simulink model "P2_SIL_Model_Diag"  (R2016a)
settings: Solver=ode2  StartTime=0.0  StopTime=Cycle_End  RelTol=1e-3
undefined symbols (not defined in the file): air, APP1_OOR, APP2_OOR, APP_Conversion_IN, APP_Mismatch, bms_inletair_temp, bms_maxchargecurrent, bms_maxdischargecurrent, BMS_Notfallkuehlung, BPP_Flt, cal, clt, ClutchEngag, CrankRequest, dcdc, eng, Engine, EngOverTemp, ENGTRQ_MSMCH_Degraded_CP, ENGTRQ_MSMCH_ErrCritical_CP, ENGTRQ_MSMCH_LimpHome_CP, EngTrqMismatch, env, ess, ESS, ESSOverTemp, fd, FFD, g, gb, Grade, IMG, KeyPos_Flt, KeyPosition, lib_APP_Conversion_IN, lib_ESS_plant_V1_2, lib_OBC_Manager, LossCAN, max_vehicle_rad_air_flow, MCUOverTemp, mot, MotDirMismatch, MotOverTemp, MotTrqMismatch, mph2kph, mph2ms, NeutralGear, obc, OBC_Manager, ParkGear, PRNDL_Flt, ReverseGear, RFD, rho, ShiftLeverPosition, sigbuilder_block, Speed, t_amb, time, tloop ... (+2)
libraries: simulink x104, EC2_libraries x12, Diagnostic x11, lib_CANerror_Detect x3, Utility x1
(part 5 of 11)

== system P2_SIL_Model_Diag/Plant Actuators/CAN/HV_CAN/BMS_Hybrid ==
  In1 : Inport
  Bus Selector : BusSelector  OutputSignals=BMS_CAN.BMS_Plugin
  Out1 : Outport
  wires:
  Bus Selector/1 -> Out1/1  "<BMS_Plugin>"
  In1/1 -> Bus Selector/1

== system P2_SIL_Model_Diag/Plant Actuators/CAN/HV_CAN/MCU ==
  In1 : Inport
  Bus Selector : BusSelector  OutputSignals=MCU_CAN
  Out1 : Outport
  wires:
  Bus Selector/1 -> Out1/1  "<MCU_CAN>"
  In1/1 -> Bus Selector/1

== system P2_SIL_Model_Diag/Plant Actuators/CAN/HV_CAN/OBC ==
  In1 : Inport
  Bus Selector : BusSelector  OutputSignals=OBC_CAN
  Out1 : Outport
  wires:
  Bus Selector/1 -> Out1/1  "<OBC_CAN>"
  In1/1 -> Bus Selector/1

== system P2_SIL_Model_Diag/Plant Actuators/CAN/VEH_CAN/BCM ==
  In1 : Inport
  Out1 : Outport
  wires:
  In1/1 -> Out1/1

== system P2_SIL_Model_Diag/Plant Actuators/CAN/VEH_CAN/EBCM ==
  In1 : Inport
  Out1 : Outport
  wires:
  In1/1 -> Out1/1

== system P2_SIL_Model_Diag/Plant Actuators/CAN/VEH_CAN/ICCM ==
  In1 : Inport
  Out1 : Outport
  wires:
  In1/1 -> Out1/1

== system P2_SIL_Model_Diag/Plant Actuators/CAN/VEH_CAN/TCM ==
  In1 : Inport
  Out1 : Outport
  wires:
  In1/1 -> Out1/1

== system P2_SIL_Model_Diag/Plant Sensors/CAN/EBCAN/BMS_Antrieb ==
  In1 : Inport
  Bus Selector : BusSelector  OutputSignals=to_EBCAN.ISO_Funktionaler_Req_All
  Out1 : Outport
  wires:
  Bus Selector/1 -> Out1/1  "<ISO_Funktionaler_Req_All>"
  In1/1 -> Bus Selector/1

== system P2_SIL_Model_Diag/Plant Sensors/CAN/EBCAN/ECM ==
  In1 : Inport
  Bus Selector : BusSelector  OutputSignals=to_EBCAN.ECM_CAN
  Out1 : Outport
  wires:
  Bus Selector/1 -> Out1/1  "<ECM_CAN>"
  In1/1 -> Bus Selector/1

== system P2_SIL_Model_Diag/Plant Sensors/CAN/HV_CAN/APM ==
  In1 : Inport
  Bus Selector : BusSelector  OutputSignals=to_HV_CAN.to_APM
  Out1 : Outport
  wires:
  In1/1 -> Bus Selector/1
  Bus Selector/1 -> Out1/1  "<to_APM>"

== system P2_SIL_Model_Diag/Plant Sensors/CAN/HV_CAN/BMS_Hybrid ==
  In1 : Inport
  Bus Selector : BusSelector  OutputSignals=to_HV_CAN.to_BMS_Hybrid
  Out1 : Outport
  wires:
  Bus Selector/1 -> Out1/1  "<to_BMS_Hybrid>"
  In1/1 -> Bus Selector/1

== system P2_SIL_Model_Diag/Plant Sensors/CAN/HV_CAN/MCU ==
  In1 : Inport
  Bus Selector : BusSelector  OutputSignals=to_HV_CAN.to_MCU
  Out1 : Outport
  wires:
  Bus Selector/1 -> Out1/1  "<to_MCU>"
  In1/1 -> Bus Selector/1

== system P2_SIL_Model_Diag/Plant Sensors/CAN/HV_CAN/OBC ==
  In1 : Inport
  Bus Selector : BusSelector  OutputSignals=to_HV_CAN.to_OBC
  Out1 : Outport
  wires:
  Bus Selector/1 -> Out1/1  "<to_OBC>"
  In1/1 -> Bus Selector/1

== system P2_SIL_Model_Diag/Plant Sensors/CAN/VEH_CAN/BCM ==
  In1 : Inport
  Bus Selector : BusSelector  OutputSignals=to_VEH_CAN.HAct_to_BCM
  Out1 : Outport
  wires:
  Bus Selector/1 -> Out1/1  "<HAct_to_BCM>"
  In1/1 -> Bus Selector/1

== system P2_SIL_Model_Diag/Plant Sensors/CAN/VEH_CAN/EBCM ==
  In1 : Inport
  Bus Selector : BusSelector  OutputSignals=to_VEH_CAN.HAct_to_EBCM
  Out1 : Outport
  wires:
  Bus Selector/1 -> Out1/1  "<HAct_to_EBCM>"
  In1/1 -> Bus Selector/1

== system P2_SIL_Model_Diag/Plant Sensors/CAN/VEH_CAN/ICCM ==
  In1 : Inport
  Bus Selector : BusSelector  OutputSignals=to_VEH_CAN.HAct_to_ICCM
  Out1 : Outport
  wires:
  Bus Selector/1 -> Out1/1  "<HAct_to_ICCM>"
  In1/1 -> Bus Selector/1

== system P2_SIL_Model_Diag/Plant Sensors/CAN/VEH_CAN/TCM ==
  In1 : Inport
  Bus Selector : BusSelector  OutputSignals=to_VEH_CAN.HAct_to_TCM
  Out1 : Outport
  wires:
  Bus Selector/1 -> Out1/1  "<HAct_to_TCM>"
  In1/1 -> Bus Selector/1

== system P2_SIL_Model_Diag/Sensors/Analog/APP Manipulation/APP1_Conversion ==
  APP1_IN : Inport
  APP1_IN_Max : Constant  Value=cal.APP1.IN_Max
  APP1_IN_Max_SC : Constant  Value=cal.APP.IN_Max_SC
  APP1_IN_Min : Constant  Value=cal.APP1.IN_Min
  Constant : Constant  Value=0
  Divide : Product  Inputs=*/
  Gain : Gain  Gain=100
  Relational Operator : RelationalOperator  Operator=>  OutDataTypeStr=boolean
  Sum1 : Sum  Inputs=|+-
  Sum2 : Sum  Inputs=|-+
  Sum3 : Sum  Inputs=|++
  Switch1 : Switch  Threshold=1
  APP1 : Outport
  OOR : Outport  Port=2
  wires:
  Sum3/1 -> Relational Operator/2
  Switch1/1 -> APP1/1
  APP1_IN_Max_SC/1 -> Sum3/2
  Relational Operator/1 -> Switch1/2, OOR/1  "APP1_SC_Fault"
  Constant/1 -> Switch1/1
  Gain/1 -> Switch1/3
  Divide/1 -> Gain/1
  Sum2/1 -> Divide/2
  Sum1/1 -> Divide/1
  APP1_IN/1 -> Relational Operator/1, Sum1/1
  APP1_IN_Max/1 -> Sum3/1, Sum2/2
  APP1_IN_Min/1 -> Sum1/2, Sum2/1

== system P2_SIL_Model_Diag/Sensors/Analog/APP Manipulation/APP2_Conversion ==
  APP2_IN : Inport
  APP1_IN_Max_SC : Constant  Value=cal.APP.IN_Max_SC
  APP2_IN_Max : Constant  Value=cal.APP2.IN_Max
  APP2_IN_Min : Constant  Value=cal.APP2.IN_Min
  Constant : Constant  Value=0
  Divide : Product  Inputs=*/
  Gain1 : Gain  Gain=100
  Relational Operator : RelationalOperator  Operator=>  OutDataTypeStr=boolean
  Sum1 : Sum  Inputs=|++
  Sum2 : Sum  Inputs=|+-
  Sum3 : Sum  Inputs=|-+
  Switch1 : Switch  Threshold=1
  APP2 : Outport
  OOR : Outport  Port=2
  wires:
  Switch1/1 -> APP2/1
  APP1_IN_Max_SC/1 -> Sum1/2
  Sum1/1 -> Relational Operator/2
  Relational Operator/1 -> Switch1/2, OOR/1  "APP2_SC_Fault"
  Constant/1 -> Switch1/1
  Gain1/1 -> Switch1/3
  Divide/1 -> Gain1/1
  Sum3/1 -> Divide/2
  Sum2/1 -> Divide/1
  APP2_IN/1 -> Relational Operator/1, Sum2/1
  APP2_IN_Max/1 -> Sum1/1, Sum3/2
  APP2_IN_Min/1 -> Sum2/2, Sum3/1

== system P2_SIL_Model_Diag/Sensors/CAN/EBCAN/BMS_Antrieb ==
  In1 : Inport
  Bus Creator : BusCreator  Inputs=2
  Bus Selector : BusSelector  OutputSignals=NMH_BMS
  ISO_Hybrid_01_Resp : Subsystem
  NMH_BMS : Subsystem
  Out1 : Outport
  wires:
  In1/1 -> Bus Selector/1
  Bus Selector/1 -> NMH_BMS/1(In1)  "<NMH_BMS>"
  NMH_BMS/1(Out1) -> Bus Creator/1
  ISO_Hybrid_01_Resp/1(Out1) -> Bus Creator/2
  Bus Creator/1 -> Out1/1

== system P2_SIL_Model_Diag/Sensors/CAN/EBCAN/CCM ==
  In1 : Inport
  ISO_Hybrid_01_Resp : Subsystem
  NMH_BMS : Subsystem
  Out1 : Outport

== system P2_SIL_Model_Diag/Sensors/CAN/EBCAN/ECM ==
  In1 : Inport
  Bus Creator : BusCreator  Inputs=7
  Bus Selector : BusSelector  OutputSignals=Sensors_to_ECM.EngActStdyStTorq_Nm,Sensors_to_ECM.EngSpd_RPM,ECM_to_Actuators.VehSpdAvgDrvn,ECM_to_Actuators.EngRunAtv,ECM_to_Actuators.EngTrqCmd,ECM_to_Actuators.Eng_Temp,ECM_to_Actuators.ECM_RollingAliveCnt
  ETEI_Engine_Torque_Status : Subsystem
  PPEI_Vehicle_Speed_and_Distance : Subsystem
  Out1 : Outport
  wires:
  In1/1 -> Bus Selector/1
  Bus Selector/1 -> ETEI_Engine_Torque_Status/1(In1)  "<EngActStdyStTorq_Nm>"
  Bus Selector/2 -> Bus Creator/2  "<EngSpd_RPM>"
  Bus Selector/3 -> PPEI_Vehicle_Speed_and_Distance/1(In1)  "<VehSpdAvgDrvn>"
  ETEI_Engine_Torque_Status/1(Out1) -> Bus Creator/1
  PPEI_Vehicle_Speed_and_Distance/1(Out1) -> Bus Creator/3
  Bus Creator/1 -> Out1/1
  Bus Selector/4 -> Bus Creator/4  "<EngRunAtv>"
  Bus Selector/5 -> Bus Creator/5  "<EngTrqCmd>"
  Bus Selector/6 -> Bus Creator/6  "<Eng_Temp>"
  Bus Selector/7 -> Bus Creator/7  "<ECM_RollingAliveCnt>"

== system P2_SIL_Model_Diag/Sensors/CAN/HV_CAN/APM ==
  In1 : Inport
  Out1 : Outport
  wires:
  In1/1 -> Out1/1

== system P2_SIL_Model_Diag/Sensors/CAN/HV_CAN/BMS_Hybrid ==
  In1 : Inport
  BMS_HYB_02 : Subsystem
  BMS_HYB_03 : Subsystem
  BMS_HYB_04 : Subsystem
  Bus Creator : BusCreator  Inputs=5
  Bus Selector : BusSelector  OutputSignals=BMS_HYB_02,BMS_HYB_04,BMS_HYB_03,RollingAliveCnt,BMS_HYB_06
  Out1 : Outport
  wires:
  In1/1 -> Bus Selector/1
  Bus Selector/1 -> BMS_HYB_02/1(In1)  "<BMS_HYB_02>"
  Bus Selector/2 -> BMS_HYB_04/1(In1)  "<BMS_HYB_04>"
  Bus Creator/1 -> Out1/1
  BMS_HYB_02/1(Out1) -> Bus Creator/1
  BMS_HYB_04/1(Out1) -> Bus Creator/2
  Bus Selector/3 -> BMS_HYB_03/1(In1)  "<BMS_HYB_03>"
  BMS_HYB_03/1(Out1) -> Bus Creator/3
  Bus Selector/4 -> Bus Creator/4  "<RollingAliveCnt>"
  Bus Selector/5 -> Bus Creator/5  "<BMS_HYB_06>"

== system P2_SIL_Model_Diag/Sensors/CAN/HV_CAN/MCU ==
  note: torque feedback should be from sensors, not MCU to Actuators
      | in this model, mot_torq_out and MotTrqFdbck are the same signals
  In1 : Inport
  Bus Creator : BusCreator  Inputs=11
  Bus Selector : BusSelector  OutputSignals=Sensors_to_MCU.mot_spd_out,Sensors_to_MCU.mot_crr_out,MCU_to _Actuator.InverterEnabled,Sensors_to_MCU.mot_volt_in,Sensors_to_MCU.mot_temp,MCU_to _Actuator.Torque_Command,MCU_to _Actuator.MotTrqFdbck,MCU_to _Actuator.EngageClutch,Sensors_to_MCU.mcu_temp,MCU_to _Actuator.RollingAliveCnt,Sensors_to_MCU.clt_plant_spd_in
  M165_Motor_Position_Info : Subsystem
  M166_Current_Info : Subsystem
  M167_Voltage_Info : Subsystem
  M170_Internal_States : Subsystem
  M172_Torque_And_Timer_Info : Subsystem
  M192_Command_Message : Subsystem
  Out1 : Outport
  wires:
  In1/1 -> Bus Selector/1
  Bus Selector/1 -> M165_Motor_Position_Info/1(In1)  "<mot_spd_out>"
  Bus Selector/2 -> M166_Current_Info/1(In1)  "<mot_crr_out>"
  Bus Selector/3 -> M170_Internal_States/1(In1)  "<InverterEnabled>"
  M165_Motor_Position_Info/1(Out1) -> Bus Creator/1
  M166_Current_Info/1(Out1) -> Bus Creator/2
  M170_Internal_States/1(Out1) -> Bus Creator/3
  Bus Creator/1 -> Out1/1
  Bus Selector/5 -> Bus Creator/5  "<mot_temp>"
  Bus Selector/6 -> M192_Command_Message/1(In1)  "<Torque_Command>"
  Bus Selector/7 -> M172_Torque_And_Timer_Info/1(In1)  "<MotTrqFdbck>"
  Bus Selector/4 -> M167_Voltage_Info/1(In1)  "<mot_volt_in>"
  M167_Voltage_Info/1(Out1) -> Bus Creator/4
  M192_Command_Message/1(Out1) -> Bus Creator/6
  M172_Torque_And_Timer_Info/1(Out1) -> Bus Creator/7
  Bus Selector/8 -> Bus Creator/8  "<EngageClutch>"
  Bus Selector/9 -> Bus Creator/9  "<mcu_temp>"
  Bus Selector/10 -> Bus Creator/10  "<RollingAliveCnt>"
  Bus Selector/11 -> Bus Creator/11  "<clt_plant_spd_in>"

== system P2_SIL_Model_Diag/Sensors/CAN/HV_CAN/OBC ==
  In1 : Inport
  Out1 : Outport
  wires:
  In1/1 -> Out1/1

== system P2_SIL_Model_Diag/Sensors/CAN/VEH_CAN/BCM ==
  In1 : Inport
  Bus Creator : BusCreator  Inputs=2
  Bus Selector : BusSelector  OutputSignals=SysPwrMd,BrkPdlPos
  PPEI_Brake_Apply_Status : Subsystem
  PPEI_Platfrom_General_Status : Subsystem
  Out1 : Outport
  wires:
  In1/1 -> Bus Selector/1
  Bus Selector/1 -> PPEI_Platfrom_General_Status/1(In1)  "<SysPwrMd>"
  Bus Selector/2 -> PPEI_Brake_Apply_Status/1(In1)  "<BrkPdlPos>"
  PPEI_Platfrom_General_Status/1(Out1) -> Bus Creator/1
  PPEI_Brake_Apply_Status/1(Out1) -> Bus Creator/2
  Bus Creator/1 -> Out1/1

== system P2_SIL_Model_Diag/Sensors/CAN/VEH_CAN/EBCM ==
  In1 : Inport
  PPEI_Chassis_General_Status_1 : Subsystem
  Out1 : Outport
  wires:
  PPEI_Chassis_General_Status_1/1(Out1) -> Out1/1

== system P2_SIL_Model_Diag/Sensors/CAN/VEH_CAN/ICCM ==
  In1 : Inport
  Out1 : Outport
  wires:
  In1/1 -> Out1/1

== system P2_SIL_Model_Diag/Sensors/CAN/VEH_CAN/TCM ==
  In1 : Inport
  Bus Creator : BusCreator  Inputs=3
  Bus Selector : BusSelector  OutputSignals=TCM_to _Actuator.TransEstGear,TCM_to _Actuator.LockupCmd,TCM_to _Actuator.TrnsShftLvrPos
  Out1 : Outport
  wires:
  In1/1 -> Bus Selector/1
  Bus Selector/1 -> Bus Creator/1  "<TransEstGear>"
  Bus Selector/2 -> Bus Creator/2  "<LockupCmd>"
  Bus Selector/3 -> Bus Creator/3  "<TrnsShftLvrPos>"
  Bus Creator/1 -> Out1/1

== system P2_SIL_Model_Diag/Camaro Plant Model/ESS/ESS/ESSThermal/LowerLimit ==
  In : Inport
  Constant : Constant  Value=Lolimit
  MinMax : MinMax  Function=max  Inputs=2
  Out : Outport
  wires:
  Constant/1 -> MinMax/2
  In/1 -> MinMax/1
  MinMax/1 -> Out/1

== system P2_SIL_Model_Diag/Camaro Plant Model/ESS/ESS/ESSThermal/LowerLimit1 ==
  In : Inport
  Constant : Constant  Value=Lolimit
  MinMax : MinMax  Function=max  Inputs=2
  Out : Outport
  wires:
  Constant/1 -> MinMax/2
  In/1 -> MinMax/1
  MinMax/1 -> Out/1

== system P2_SIL_Model_Diag/Camaro Plant Model/ESS/ESS/LoadCharacteristics/LowerLimit1 ==
  In : Inport
  Constant : Constant  Value=Lolimit
  MinMax : MinMax  Function=max  Inputs=2
  Out : Outport
  wires:
  Constant/1 -> MinMax/2
  In/1 -> MinMax/1
  MinMax/1 -> Out/1

== system P2_SIL_Model_Diag/Camaro Plant Model/ESS/ESS/LoadCharacteristics/LowerLimit2 ==
  In : Inport
  Constant : Constant  Value=Lolimit
  MinMax : MinMax  Function=max  Inputs=2
  Out : Outport
  wires:
  Constant/1 -> MinMax/2
  In/1 -> MinMax/1
  MinMax/1 -> Out/1

== system P2_SIL_Model_Diag/Camaro Plant Model/ESS/ESS/LoadCharacteristics/SOC Calculation ==
  Current : Inport
  3600*nominal battery capacity : Constant  Value=3600*ess.plant.init.batcap
  Sum3 : Sum  Inputs=|++
  To Workspace : ToWorkspace  VariableName=ess_soc_percent_hist  SampleTime=-1
      settings: Decimation=WORKSPACE_DECIMATION
  i/3600C : Product  Inputs=*/  RndMeth=Zero
  soc previous state : Memory  X0=ess.plant.init.initial_soc/100  InheritSampleTime=on
  soc limits : Saturate  UpperLimit=1  LowerLimit=0
  tloop : Gain  Gain=tloop
  to % : Gain  Gain=100
  SOC : Outport
  wires:
  3600*nominal battery capacity/1 -> i/3600C/2  "As"
  i/3600C/1 -> tloop/1  "dSOC/s"
  to %/1 -> To Workspace/1
  soc limits/1 -> to %/1, SOC/1, soc previous state/1
  tloop/1 -> Sum3/1  "dSOC"
  Sum3/1 -> soc limits/1
  soc previous state/1 -> Sum3/2  "soc"
  Current/1 -> i/3600C/1  "A"

== system P2_SIL_Model_Diag/Camaro Plant Model/ESS/Soft BMS/Energy Consumption/Divide by zero ==
  In1 : Inport
  Compare To Constant : simulink/Logic and Bit Operations/Compare To Constant  relop===  const=0  OutDataTypeStr=boolean
  Constant1 : Constant  Value=eps
  Switch2 : Switch  Criteria=u2 > Threshold
  Out1 : Outport
  wires:
  Constant1/1 -> Switch2/1
  Compare To Constant/1 -> Switch2/2
  In1/1 -> Switch2/3, Compare To Constant/1
  Switch2/1 -> Out1/1

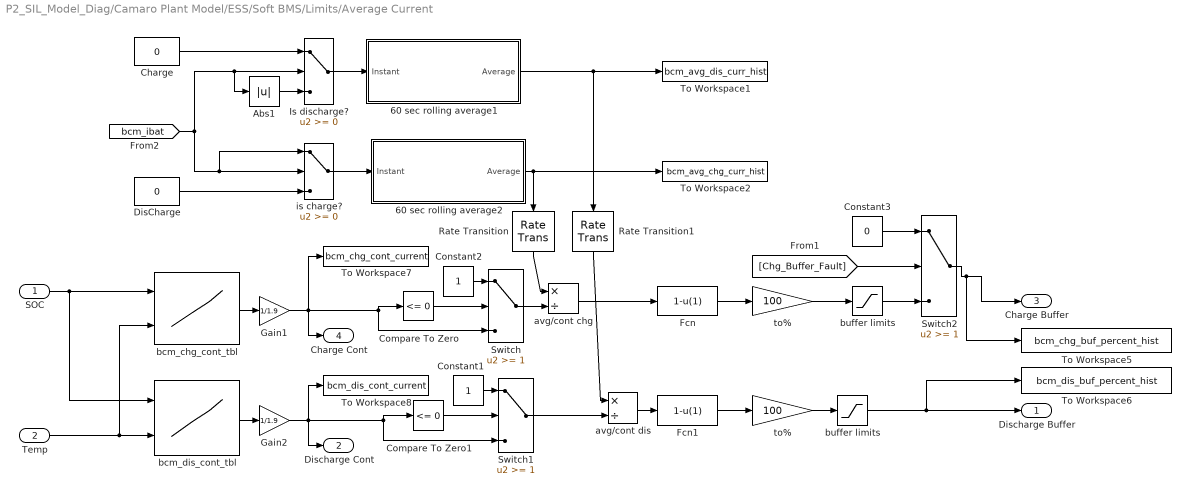
== system P2_SIL_Model_Diag/Camaro Plant Model/ESS/Soft BMS/Limits/Average Current ==
  SOC : Inport
  Temp : Inport  Port=2
  60 sec rolling average1 : Subsystem
  60 sec rolling average2 : Subsystem
  Abs1 : Abs
  Charge : Constant  Value=0
  Compare To Zero : simulink/Logic and Bit Operations/Compare To Zero  relop=<=  OutDataTypeStr=boolean
  Compare To Zero1 : simulink/Logic and Bit Operations/Compare To Zero  relop=<=  OutDataTypeStr=boolean
  Constant1 : Constant
  Constant2 : Constant
  Constant3 : Constant  Value=0
  DisCharge : Constant  Value=0
  Fcn : Fcn  Expr=1-u(1)
  Fcn1 : Fcn  Expr=1-u(1)
  Gain1 : Gain  Gain=1/1.9
  Gain2 : Gain  Gain=1/1.9
  Is discharge? : Switch
  Rate Transition : RateTransition
  Rate Transition1 : RateTransition
  Switch : Switch  Threshold=1
  Switch1 : Switch  Threshold=1
  Switch2 : Switch  Threshold=1
  To Workspace1 : ToWorkspace  VariableName=bcm_avg_dis_curr_hist  SampleTime=-1
      settings: Decimation=WORKSPACE_DECIMATION
  To Workspace2 : ToWorkspace  VariableName=bcm_avg_chg_curr_hist  SampleTime=-1
      settings: Decimation=WORKSPACE_DECIMATION
  To Workspace5 : ToWorkspace  VariableName=bcm_chg_buf_percent_hist  SampleTime=-1
      settings: Decimation=WORKSPACE_DECIMATION
  To Workspace6 : ToWorkspace  VariableName=bcm_dis_buf_percent_hist  SampleTime=-1
      settings: Decimation=WORKSPACE_DECIMATION
  To Workspace7 : ToWorkspace  VariableName=bcm_chg_cont_current  SampleTime=-1
      settings: Decimation=WORKSPACE_DECIMATION
  To Workspace8 : ToWorkspace  VariableName=bcm_dis_cont_current  SampleTime=-1
      settings: Decimation=WORKSPACE_DECIMATION
  avg/cont chg : Product  Inputs=*/  RndMeth=Zero
  avg/cont dis : Product  Inputs=*/  RndMeth=Zero
  bcm_chg_cont_tbl : Lookup2D  RowIndex=ess.plant.init.limit.idx1_soc  ColumnIndex=ess.plant.init.limit.idx2_temp  Table=ess.plant.init.max_cont_charge
  bcm_dis_cont_tbl : Lookup2D  RowIndex=ess.plant.init.limit.idx1_soc  ColumnIndex=ess.plant.init.limit.idx2_temp  Table=ess.plant.init.max_cont_discharge
  buffer limits : Saturate  UpperLimit=100  LowerLimit=0
  "buffer limits " : Saturate  UpperLimit=100  LowerLimit=0
  is charge? : Switch
  to% : Gain  Gain=100
  "to% " : Gain  Gain=100
  Discharge Buffer : Outport
  Discharge Cont : Outport  Port=2
  Charge Buffer : Outport  Port=3
  Charge Cont : Outport  Port=4
  wires:
  [Chg_Buffer_Fault] -> Switch2/2
  Constant3/1 -> Switch2/1
  Switch2/1 -> To Workspace5/1, Charge Buffer/1
  buffer limits/1 -> Switch2/3
  Temp/1 -> bcm_dis_cont_tbl/2, bcm_chg_cont_tbl/2
  to%/1 -> buffer limits/1
  "to% "/1 -> "buffer limits "/1
  Fcn1/1 -> "to% "/1
  Fcn/1 -> to%/1
  avg/cont dis/1 -> Fcn1/1
  avg/cont chg/1 -> Fcn/1
  60 sec rolling average2/1(Average) -> To Workspace2/1, Rate Transition/1
  60 sec rolling average1/1(Average) -> To Workspace1/1, Rate Transition1/1
  is charge?/1 -> 60 sec rolling average2/1(Instant)
  Is discharge?/1 -> 60 sec rolling average1/1(Instant)
  DisCharge/1 -> is charge?/3
  Abs1/1 -> Is discharge?/3
  Charge/1 -> Is discharge?/1
  [bcm_ibat] -> is charge?/1, is charge?/2, Abs1/1, Is discharge?/2
  SOC/1 -> bcm_chg_cont_tbl/1, bcm_dis_cont_tbl/1
  Compare To Zero/1 -> Switch/2
  Constant2/1 -> Switch/1
  Switch/1 -> avg/cont chg/2
  bcm_chg_cont_tbl/1 -> Gain1/1
  Compare To Zero1/1 -> Switch1/2
  Constant1/1 -> Switch1/1
  Switch1/1 -> avg/cont dis/2
  bcm_dis_cont_tbl/1 -> Gain2/1
  "buffer limits "/1 -> To Workspace6/1, Discharge Buffer/1
  Gain1/1 -> To Workspace7/1, Compare To Zero/1, Switch/3, Charge Cont/1
  Gain2/1 -> Discharge Cont/1, Compare To Zero1/1, Switch1/3, To Workspace8/1
  Rate Transition/1 -> avg/cont chg/1
  Rate Transition1/1 -> avg/cont dis/1

== system P2_SIL_Model_Diag/Camaro Plant Model/ESS/Soft BMS/Limits/Derate ==
  Current Limit : Inport
  Buffer : Inport  Port=2
  Cont Current : Inport  Port=3
  100A/sec : Gain  Gain=100*tloop
  Compare To Zero2 : simulink/Logic and Bit Operations/Compare To Zero  relop=<=  OutDataTypeStr=boolean
  Gain : Gain  Gain=-1
  Memory1 : Memory
  MinMax : MinMax  Function=max  Inputs=2
  StepTm[sec] : Constant  Value=tloop
  Sum : Sum  Inputs=|++
  Sum1 : Sum  Inputs=|-+
  Switch1 : Switch  Threshold=1
  Derate : Outport
  wires:
  Sum/1 -> Memory1/1, 100A/sec/1
  Switch1/1 -> Sum/1
  StepTm[sec]/1 -> Switch1/1
  Memory1/1 -> Gain/1, Sum/2
  Gain/1 -> Switch1/3
  Buffer/1 -> Compare To Zero2/1
  Compare To Zero2/1 -> Switch1/2
  100A/sec/1 -> Sum1/1
  Sum1/1 -> MinMax/1
  Current Limit/1 -> Sum1/2
  MinMax/1 -> Derate/1
  Cont Current/1 -> MinMax/2

== system P2_SIL_Model_Diag/Camaro Plant Model/ESS/Soft BMS/Limits/Derate2 ==
  Buffer : Inport
  Cont Current : Inport  Port=2
  Current Limit : Inport  Port=3
  100A/sec : Gain  Gain=100*tloop
  Compare To Zero2 : simulink/Logic and Bit Operations/Compare To Zero  relop=<=  OutDataTypeStr=boolean
  Gain : Gain  Gain=-1
  Memory1 : Memory
  MinMax : MinMax  Function=max  Inputs=2
  StepTm[sec] : Constant  Value=tloop
  Sum : Sum  Inputs=|++
  Sum1 : Sum  Inputs=|-+
  Switch1 : Switch  Threshold=1
  Derate : Outport
  wires:
  Cont Current/1 -> MinMax/2
  MinMax/1 -> Derate/1
  Current Limit/1 -> Sum1/2
  Sum1/1 -> MinMax/1
  100A/sec/1 -> Sum1/1
  Compare To Zero2/1 -> Switch1/2
  Buffer/1 -> Compare To Zero2/1
  Gain/1 -> Switch1/3
  Memory1/1 -> Sum/2, Gain/1
  StepTm[sec]/1 -> Switch1/1
  Switch1/1 -> Sum/1
  Sum/1 -> 100A/sec/1, Memory1/1

== system P2_SIL_Model_Diag/Camaro Plant Model/ICE Simple1/Engine Plant Modified/Core Engine/Crank Process/function ==
  EngSpd : Inport
  f : TriggerPort  TriggerType=function-call  VariantControl=Variant
      settings: CopyFcn=Stateflow.SLINSF.SimulinkMan.removeBlockPreDeleteFcn  PreDeleteFcn=Stateflow.SLINSF.SimulinkMan.unsafePredeleteFcn
  1-D Lookup Table : Lookup_n-D  NumberOfTableDimensions=1  BreakpointsForDimension1=[0 50 120 210 300 320 340 350 400]  Table="[90 90 90 10 5 5  5 5 5]"  InternalRulePriority=Speed  RndMeth=Simplest  InputSameDT=on
  Sine Wave : Sin  Amplitude=20  Frequency=41.88
  Sum : Sum
  CrankTrq : Outport
  wires:
  1-D Lookup Table/1 -> Sum/1
  EngSpd/1 -> 1-D Lookup Table/1
  Sum/1 -> CrankTrq/1
  Sine Wave/1 -> Sum/2

== system P2_SIL_Model_Diag/Camaro Plant Model/ICE Simple1/Engine Plant Modified/Core Engine/EngEfficiency ==
  note: Mechanical Power [W]
  Torque : Inport
  Speed : Inport  Port=2
  Fuel Consumption : Inport  Port=3
  Divide by Zero Fix : Subsystem
  Divide_by_Zero_Fix1 : EC2_libraries/Divide_by_Zero_Fix  Commented=on
  From1 : From  Commented=on  GotoTag=Wh_out
  From2 : From  Commented=on  GotoTag=Wh_in
  Goto1 : Goto  Commented=on  GotoTag=Wh_out
  Goto2 : Goto  Commented=on  GotoTag=Wh_in
  Integrator1 : Integrator  Commented=on  LimitOutput=on  LowerSaturationLimit=0
  Integrator2 : Integrator  Commented=on  LimitOutput=on  LowerSaturationLimit=0
  OnlyPositiveEnergy : Saturate  Commented=on  UpperLimit=inf  LowerLimit=0
  Percentage Efficiency : Gain  Gain=100
  Product : Product  RndMeth=Zero
  Scope : Scope  NumInputPorts=2
  Specific Energy LHV in J/kg : Gain  Gain=Engine.Fuel.Lower_Heating_Value/1000
  Sum : Sum  Inputs=-+
  To Workspace7 : ToWorkspace  Commented=on  VariableName=eng_Wh_pos_eff_hist  SampleTime=-1
      settings: Decimation=WORKSPACE_DECIMATION
  engine_efficiency : Scope
  limit_efficiency[0-100%] : Saturate  UpperLimit=100  LowerLimit=0
  PowerLoss : Outport
  wires:
  limit_efficiency[0-100%]/1 -> engine_efficiency/1
  Sum/1 -> PowerLoss/1  "Losses [W]"
  Fuel Consumption/1 -> Specific Energy LHV in J/kg/1
  Specific Energy LHV in J/kg/1 -> Divide by Zero Fix/2(Divide), Sum/2, Integrator2/1, Scope/2  "Thermal Power [W]"
  Torque/1 -> Product/2  "Nm"
  Speed/1 -> Product/1  "rpm"
  Percentage Efficiency/1 -> limit_efficiency[0-100%]/1  "Efficiency [%]"
  Divide by Zero Fix/1(Output) -> Percentage Efficiency/1
  Product/1 -> Scope/1, Divide by Zero Fix/1(Multiply), OnlyPositiveEnergy/1, Sum/1  "wer [W]"
  Divide_by_Zero_Fix1/1 -> To Workspace7/1
  From1/1 -> Divide_by_Zero_Fix1/1
  From2/1 -> Divide_by_Zero_Fix1/2
  Integrator1/1 -> Goto1/1
  OnlyPositiveEnergy/1 -> Integrator1/1
  Integrator2/1 -> Goto2/1

== system P2_SIL_Model_Diag/Camaro Plant Model/ICE Simple1/Engine Plant Modified/Core Engine/EngineThermal ==
  note: Temp Delta C deg
  PowerLoss : Inport
  Divide : Product  Inputs=*/
  Divide1 : Product  Inputs=**
  Engine Mass : Constant  Value=Engine.Mass
  Memory : Memory  X0=Engine.Init_T_amb
  Memory1 : Memory
  Product : Product  RndMeth=Zero
  Specific Heat Cap Aluminum : Constant  Value=Engine.Specific_Heat
  Sum : Sum  Inputs=|++
  Sum1 : Sum  Inputs=|+-
  tloop : Constant  Value=0.01
  Temp[degC] : Outport
  tag scope: Heat_Transfer_Eng=global
  wires:
  Memory1/1 -> Sum1/2
  Divide1/1 -> Divide/1  "J"
  Sum1/1 -> Divide1/2
  Memory/1 -> Sum/2
  PowerLoss/1 -> Sum1/1, [Heat_Transfer_Eng]  "J/s"
  Engine Mass/1 -> Product/1  "kg"
  Specific Heat Cap Aluminum/1 -> Product/2  "J/kg*K"
  Product/1 -> Divide/2
  Sum/1 -> Memory/1, Temp[degC]/1
  Divide/1 -> Sum/1
  tloop/1 -> Divide1/1
  [Heat_Reject_Eng] -> Memory1/1

== system P2_SIL_Model_Diag/Camaro Plant Model/ICE Simple1/Engine Plant Modified/Core Engine/engine filter ==
  cmd : Inport
  trq : Inport  Port=2
  Interval Test : simulink/Logic and Bit Operations/Interval Test  IntervalClosedRight=on  uplimit=0.02  IntervalClosedLeft=on  lowlimit=-0.02  OutDataTypeStr=boolean
  Switch : Switch  Threshold=0.5
  engine time response : TransferFcn  Denominator=[0.3 1]
  filtered : Outport
  wires:
  Switch/1 -> filtered/1
  cmd/1 -> Interval Test/1
  Interval Test/1 -> Switch/2
  engine time response/1 -> Switch/3
  trq/1 -> engine time response/1, Switch/1

== system P2_SIL_Model_Diag/Camaro Plant Model/ICE Simple1/Engine Plant Modified/Radiator/Divide by Zero Fix ==
  Multiply : Inport
  Divide : Inport  Port=2
  Compare To Zero : simulink/Logic and Bit Operations/Compare To Zero  relop===  OutDataTypeStr=boolean
  Constant1 : Constant  Value=0
  Constant2 : Constant
  Product2 : Product  Inputs=/*  SaturateOnIntegerOverflow=on  InputSameDT=on  OutDataTypeStr=Inherit: Same as first input
  Switch : Switch  Threshold=1
  Switch1 : Switch  Threshold=1
  Output : Outport
  wires:
  Multiply/1 -> Product2/2
  Switch1/1 -> Output/1
  Constant1/1 -> Switch1/1
  Product2/1 -> Switch1/3
  Switch/1 -> Product2/1
  Divide/1 -> Switch/3, Compare To Zero/1
  Constant2/1 -> Switch/1
  Compare To Zero/1 -> Switch1/2, Switch/2

== system P2_SIL_Model_Diag/Camaro Plant Model/ICE Simple1/Soft ECM/Fuel Consumption/Divide by Zero Fix ==
  Divide : Inport
  Multiply : Inport  Port=2
  Compare To Zero : simulink/Logic and Bit Operations/Compare To Zero  relop===  OutDataTypeStr=boolean
  Constant1 : Constant  Value=0
  Constant2 : Constant
  Product2 : Product  Inputs=/*  SaturateOnIntegerOverflow=on  InputSameDT=on  OutDataTypeStr=Inherit: Same as first input
  Switch : Switch  Threshold=1
  Switch1 : Switch  Threshold=1
  Output : Outport
  wires:
  Multiply/1 -> Product2/2
  Switch1/1 -> Output/1
  Constant1/1 -> Switch1/1
  Product2/1 -> Switch1/3
  Switch/1 -> Product2/1
  Divide/1 -> Compare To Zero/1, Switch/3
  Constant2/1 -> Switch/1
  Compare To Zero/1 -> Switch1/2, Switch/2

== system P2_SIL_Model_Diag/Camaro Plant Model/ICE Simple1/Soft ECM/Fuel Consumption/Divide by Zero Fix1 ==
  Divide : Inport
  Multiply : Inport  Port=2
  Compare To Zero : simulink/Logic and Bit Operations/Compare To Zero  relop===  OutDataTypeStr=boolean
  Constant1 : Constant  Value=0
  Constant2 : Constant
  Product2 : Product  Inputs=/*  SaturateOnIntegerOverflow=on  InputSameDT=on  OutDataTypeStr=Inherit: Same as first input
  Switch : Switch  Threshold=1
  Switch1 : Switch  Threshold=1
  Output : Outport
  wires:
  Compare To Zero/1 -> Switch/2, Switch1/2
  Constant2/1 -> Switch/1
  Divide/1 -> Compare To Zero/1, Switch/3
  Switch/1 -> Product2/1
  Product2/1 -> Switch1/3
  Constant1/1 -> Switch1/1
  Switch1/1 -> Output/1
  Multiply/1 -> Product2/2

== system P2_SIL_Model_Diag/Camaro Plant Model/IMG/IMG Plant/Clutch/Inertia Calculaion ==
  inertia in : Inport
  lockup cmd : Inport  Port=2
  Cluth out Inertia : Constant  Value=clt.plant.init.inertia
  Sum5 : Sum  Inputs=|++  SaturateOnIntegerOverflow=on  InputSameDT=on  OutDataTypeStr=Inherit: Same as first input
  Switch2 : Switch  Threshold=eps  SaturateOnIntegerOverflow=on  InputSameDT=on
  clutch out inertia : Outport
  clutch in inertia : Outport  Port=2
  wires:
  Cluth out Inertia/1 -> Sum5/2, Switch2/3
  inertia in/1 -> clutch in inertia/1, Sum5/1
  lockup cmd/1 -> Switch2/2
  Sum5/1 -> Switch2/1
  Switch2/1 -> clutch out inertia/1

== system P2_SIL_Model_Diag/Camaro Plant Model/IMG/IMG Plant/Clutch/Speed Calculaion ==
  clutch out spd : Inport
  clutch in inertia : Inport  Port=2
  lockup cmd : Inport  Port=3
  clutch in trq : Inport  Port=4
  Clutch Accel : Subsystem  mask(Division){}
      mask Display: disp('/')
  Memory : Memory
  Only Positive : Saturate  UpperLimit=inf  LowerLimit=0
  Slip speed integrator : Subsystem  mask(Resettable integrator){init=clt.plant.init.spd_idle}
      mask prompts: init "Initial value:"
      mask help: Integrates first input. If second input is not zero, integration stops and state is set to third input.
      mask Help: RESETTABLE INTEGRATOR  The resettable integrator is a masked function. This block has same functionality as the built-in RESET INTEGRATOR except that when input 2 is non-zero, the block stops integration.
  Sum : Sum  Inputs=|+-
  input shaft free wheeling losses : Subsystem
  clutch in spd : Outport
  wires:
  Only Positive/1 -> Memory/1
  Slip speed integrator/1(Output) -> input shaft free wheeling losses/1(input shaft speed), Only Positive/1
  Clutch Accel/1(x\y) -> Slip speed integrator/1(Integrand)
  lockup cmd/1 -> Slip speed integrator/2(Control)
  clutch out spd/1 -> Slip speed integrator/3(Reset value)
  clutch in inertia/1 -> Clutch Accel/1(y)
  clutch in trq/1 -> Sum/1
  Memory/1 -> clutch in spd/1
  input shaft free wheeling losses/1(input shaft decel) -> Sum/2
  Sum/1 -> Clutch Accel/2(x)

== system P2_SIL_Model_Diag/Camaro Plant Model/IMG/IMG Plant/Clutch/Torque Calculaion ==
  note: mode 0 = unlock
      | mode 1 = lock up
  lockup cmd : Inport
  input trq : Inport  Port=2
  Constant7 : Constant  Value=2*pi/3
  Engagement pressure : Constant  Value=clt.plant.init.pressure  VectorParams1D=off
  Kinetic friction constant : Constant  Value=clt.plant.init.friction_coeff
  Logical Operator : Logic  Operator=NOT  AllPortsSameDT=off  OutDataTypeStr=boolean
  MinMax : MinMax  Inputs=2
  R_inner^3 : Gain  Gain=clt.plant.init.radius.inner*clt.plant.init.radius.inner*clt.plant.init.radius.inner
  R_outer^3 : Gain  Gain=clt.plant.init.radius.outer*clt.plant.init.radius.outer*clt.plant.init.radius.outer
  Rate Limiter : RateLimiter  RisingSlewLimit=2e6  FallingSlewLimit=-2e6  SampleTimeMode=inherited
  Sum : Sum  Inputs=-+
  Switch : Switch  Threshold=1
  Switch1 : Switch  Threshold=1
  Switch2 : Switch  Threshold=1
  constant1 : Constant  Value=0
  constant2 : Constant  Value=0
  lockup cmd1 : InportShadow
  torque capacity : Product  Inputs=3  SaturateOnIntegerOverflow=on  InputSameDT=on  OutDataTypeStr=Inherit: Same as first input
  clutch out trq : Outport
  wires:
  Sum/1 -> torque capacity/3
  Kinetic friction constant/1 -> torque capacity/2
  torque capacity/1 -> MinMax/1
  lockup cmd/1 -> Logical Operator/1, Switch2/3
  MinMax/1 -> Switch1/1
  Constant7/1 -> R_outer^3/1, R_inner^3/1
  R_inner^3/1 -> Sum/1
  R_outer^3/1 -> Sum/2
  Engagement pressure/1 -> Switch/1
  constant1/1 -> Switch/3
  Rate Limiter/1 -> torque capacity/1  "P"
  Switch/1 -> Rate Limiter/1
  lockup cmd1/1 -> Switch1/2
  input trq/1 -> MinMax/2
  Switch1/1 -> clutch out trq/1
  constant2/1 -> Switch1/3
  [ClutchEngagFlt] -> Switch2/2
  Logical Operator/1 -> Switch2/1
  Switch2/1 -> Switch/2

== system P2_SIL_Model_Diag/Camaro Plant Model/IMG/IMG Plant/Electric Machine/Calculate Mot Efficiency, MotPwrMech, and, MotPwrElec ==
  note: Pelec_req = Pmech_req*Eff^k,
      | k = -1 if Trq >= 0,
      | k = 1 if Trq < 0
  MotSpd : Inport
  MotTrqAct : Inport  Port=2
  -1 : Gain  Gain=8
  "-1 when + 1 when - " : Gain  Gain=-1
  -2 : Gain  Gain=tloop
  2-D Lookup Table : Lookup_n-D  BreakpointsForDimension1=mot.plant.init.eff_trq.idx2_trq  BreakpointsForDimension2=mot.plant.init.eff_trq.idx1_spd  Table=mot.plant.init.eff_trq.map  InternalRulePriority=Speed  RndMeth=Simplest  InputSameDT=on
  Abs{,1..3} (4 alike) : Abs
  Add : Sum  Inputs=-+
  Add1 : Sum  Inputs=+-
  Add2 : Sum
  Constant : Constant  Value=mot.plant.init.mcu_eff
  Constant1 : Constant  Value=mot.plant.init.mcu_mass
  Constant2 : Constant  Value=mot.plant.init.specific_heat
  Divide : Product  Inputs=*/
  Gain : Gain  Gain=3
  Gain2 : Gain  Gain=1/100
  Lower Limit : Subsystem  mask{Lolimit=t_amb+20}
      mask prompts: Lolimit "Lower Limit"
  MCU_WEGPmp : Constant  Value=0
  Math Function1 : Math  Operator=pow  SaturateOnIntegerOverflow=on
  Memory : Memory
  Memory1 : Memory
  Product{,1..3} (4 alike) : Product
  Sign : Signum
  Switch : Switch  Threshold=1
  rad/s to rpm : Gain  Gain=30/pi
  Losses : Outport
  MotPwrElec : Outport  Port=2
  MCU_Temp : Outport  Port=3
  wires:
  rad/s to rpm/1 -> Abs1/1
  Abs1/1 -> 2-D Lookup Table/2
  Sign/1 -> "-1 when + 1 when - "/1
  Abs/1 -> 2-D Lookup Table/1
  Gain2/1 -> Math Function1/1
  2-D Lookup Table/1 -> Gain2/1
  Product1/1 -> Product2/1, Add/2, MotPwrElec/1  "MotPwrElec"
  Product/1 -> Add/1, Product1/1  "MotPwrMech"
  MotTrqAct/1 -> Memory/1, Product/1, Abs/1
  MotSpd/1 -> Product/2, rad/s to rpm/1
  "-1 when + 1 when - "/1 -> Math Function1/2
  Abs2/1 -> Losses/1
  Add/1 -> Abs2/1
  Math Function1/1 -> Product1/2
  Memory/1 -> Sign/1
  Constant/1 -> Product2/2
  Product2/1 -> Abs3/1
  Abs3/1 -> Add1/1
  MCU_WEGPmp/1 -> -1/1
  Add1/1 -> -2/1
  -1/1 -> Add1/2
  -2/1 -> Divide/1
  Constant1/1 -> Product3/1
  Constant2/1 -> Product3/2
  Product3/1 -> Divide/2
  Divide/1 -> Add2/1
  Memory1/1 -> Add2/2
  Add2/1 -> Lower Limit/1(In1)
  Lower Limit/1(Out1) -> Switch/3, Gain/1, Memory1/1
  [MCUOverTemp] -> Switch/2
  Gain/1 -> Switch/1
  Switch/1 -> MCU_Temp/1

== system P2_SIL_Model_Diag/Camaro Plant Model/IMG/IMG Plant/Electric Machine/MotTrqExcessTrigger ==
  In1 : Inport
  Bias : Bias  Bias=55
  Bias1 : Bias  Bias=25
  Multiport Switch : MultiPortSwitch  DataPortOrder=Zero-based contiguous
  Signal Builder : Subsystem  Tag=STV Subsys  LoadFcn=sigbuilder_block('load');  StartFcn=sigbuilder_block('start');  StopFcn=sigbuilder_block('stop');  ClipboardFcn=sigbuilder_block('clipboard');  mask(Sigbuilder block){}
      mask help: Simulink:masks:SigbuilderBlock_MD
      mask init:
      | if ~strcmp(get_param(bdroot(gcbh),'SimulationStatus'),'stopped') tuvar = sigbuilder_block('maskInit'); end
      settings: CopyFcn=sigbuilder_block('copy');  DeleteFcn=sigbuilder_block('delete');  ModelCloseFcn=sigbuilder_block('modelClose');  PreSaveFcn=sigbuilder_block('preSave');  PauseFcn=sigbuilder_block('pause');  ContinueFcn=sigbuilder_block('continue');  NameChangeFcn=sigbuilder_block('namechange');  OpenFcn=sigbuilder_block('open',[148.2 70.2 550.2 400.2 ]);  CloseFcn=sigbuilder_block('close');
      mask Display: plot(0, 0, 100, 100,[2, 2, 32, 32, 2], [68, 8, 8, 68, 68],[32, 2], [38, 38], [32, 19, 2],[53, 60, 44], [32, 17, 17, 2],[16, 16, 31, 31]);txt = getActiveGroup(gcbh);text(2, 100, txt,'verticalAlignment', 'top');
  Out1 : Outport
  tag scope: MotTrqExcessTrig=global
  wires:
  Multiport Switch/1 -> Out1/1
  Bias/1 -> Multiport Switch/4
  In1/1 -> Multiport Switch/2, Bias/1, Bias1/1
  Bias1/1 -> Multiport Switch/3
  Signal Builder/1(Signal 1) -> [MotTrqExcessTrig], Multiport Switch/1

== system P2_SIL_Model_Diag/Camaro Plant Model/IMG/IMG Plant/Electric Machine/Thermal ==
  Losses : Inport
  Ground : Ground
  Terminator : Terminator
  mot_temp_C : Outport
  wires:
  Losses/1 -> Terminator/1  "[W]"
  Ground/1 -> mot_temp_C/1

== system P2_SIL_Model_Diag/Camaro Plant Model/IMG/IMG Plant/Electric Machine/Torque Calculation ==
  MotSpd : Inport
  MotTrqCmd : Inport  Port=2
  Abs : Abs
  Abs1 : Abs
  MinMax : MinMax  Inputs=2
  Product : Product
  Sign : Signum
  electric machine filter : Subsystem
  "max torque " : Subsystem
  mot_trq_out : Outport
  wires:
  "max torque "/1(max torque) -> Abs1/1
  MotSpd/1 -> "max torque "/2(speed)
  Sign/1 -> Product/1
  MinMax/1 -> Product/2
  Abs/1 -> MinMax/1
  Abs1/1 -> MinMax/2
  electric machine filter/1(filtered) -> mot_trq_out/1
  MotTrqCmd/1 -> "max torque "/1(cmd), Sign/1, Abs/1
  Product/1 -> electric machine filter/1(trq)

== system P2_SIL_Model_Diag/Camaro Plant Model/IMG/IMG Plant/Electric Machine/non-zero division ==
  note: original idea from Phil Sharer - ANL
      | original formula: u[1]\(u[2]+eps)*(u[2]!=0)
      | changes done by Gerald ZINI (dgey) - ANL (05\02\2001)
  note: (u[2]==0) is true then returns 1, thus (u[2]+(u[2]==0)) is equal to 0+1=1
  note: if u[2] == 0, then output == 0:
  note: (u[2]!=0) is false then returns 0
  note: and finally, the expression is: (u[1] \ 1) * 0 = 0
  note: (u[2]==0) is false then returns 0, thus (u[2]+(u[2]==0)) is equal to u[2]+0=u[2]
  note: if u[2] != 0, then output == u[1]\u[2]:
  note: (u[2]!=0) is true then returns 1
  note: and finally, the expression is: (u[1] \ u[2]) * 1 = u[1] \ u[2]
  In1 : Inport
  In2 : Inport  Port=2
  Fcn : Fcn  Expr=u[1]/(u[2]+(u[2]==0))*(u[2]!=0)
  Mux : Mux  Inputs=2
  Out1 : Outport
  wires:
  Mux/1 -> Fcn/1
  In1/1 -> Mux/1
  Fcn/1 -> Out1/1
  In2/1 -> Mux/2

== system P2_SIL_Model_Diag/Camaro Plant Model/IMG/Soft MCU/Torque Calculation/max torque  ==
  Req : Inport
  speed : Inport  Port=2
  torque : Inport  Port=3
  2-D Lookup Table : Lookup_n-D  Commented=on  BreakpointsForDimension1=mot.plant.init.eff_trq.idx2_trq  BreakpointsForDimension2=mot.plant.init.eff_trq.idx1_spd  Table=mot.plant.init.eff_trq.map  InternalRulePriority=Speed  RndMeth=Simplest  InputSameDT=on
  Abs : Abs  SaturateOnIntegerOverflow=on
  Abs1 : Abs  Commented=on
  Abs2 : Abs  Commented=on
  Constant : Constant  Commented=on  Value=84500
  Cont trq max - Motoring : Lookup  InputValues=mot.plant.init.motor.trq_cont.idx1_spd  Table=mot.plant.init.motor.trq_cont.map  LookUpMeth=Interpolation-Use End Values  SaturateOnIntegerOverflow=on
  Cont trq max - Regen : Lookup  InputValues=mot.plant.init.regen.trq_cont.idx1_spd  Table=mot.plant.init.regen.trq_cont.map  LookUpMeth=Interpolation-Use End Values  SaturateOnIntegerOverflow=on
  Divide : Product  Commented=on  Inputs=**/
  Divide by zero : Subsystem  Commented=on
  Gain2 : Gain  Commented=on  Gain=1/100
  Heat index : Subsystem
  Memory : Memory
  Peak trq max - Motoring : Lookup  Commented=on  InputValues=mot.plant.init.regen.trq_max.idx1_spd  Table=mot.plant.init.motor.trq_max.map  LookUpMeth=Interpolation-Use End Values  SaturateOnIntegerOverflow=on
  Peak trq max - Motoring1 : Lookup  InputValues=mot.plant.init.regen.trq_max.idx1_spd  Table=mot.plant.init.motor.trq_max.map  LookUpMeth=Interpolation-Use End Values  SaturateOnIntegerOverflow=on
  Peak trq max - Regen : Lookup  InputValues=mot.plant.init.regen.trq_max.idx1_spd  Table=mot.plant.init.regen.trq_max.map  LookUpMeth=Interpolation-Use End Values  SaturateOnIntegerOverflow=on
  Product2 : Product  SaturateOnIntegerOverflow=on  InputSameDT=on  OutDataTypeStr=Inherit: Same as first input
  Product3 : Product  SaturateOnIntegerOverflow=on  InputSameDT=on  OutDataTypeStr=Inherit: Same as first input
  Product5 : Product  SaturateOnIntegerOverflow=on  InputSameDT=on  OutDataTypeStr=Inherit: Same as first input
  RPM to rad/s : Gain  Commented=on  Gain=pi/30
  Sign : Signum
  Sum : Sum  SaturateOnIntegerOverflow=on  InputSameDT=on  OutDataTypeStr=Inherit: Same as first input
  Sum1 : Sum  Inputs=-+  SaturateOnIntegerOverflow=on  InputSameDT=on  OutDataTypeStr=Inherit: Same as first input
  Switch : Switch  SaturateOnIntegerOverflow=on
  Switch1 : Switch  SaturateOnIntegerOverflow=on
  cst : Constant
  rad/s  to RPM : Gain  Gain=30/pi
  max torque : Outport
  wires:
  Heat index/1(Heat index) -> Product2/2, Sum1/1
  cst/1 -> Sum1/2
  Product3/1 -> Sum/2
  Sum1/1 -> Product3/1
  Product2/1 -> Sum/1
  Switch1/1 -> Product3/2
  Switch/1 -> Heat index/1(cont torque), Product2/1
  Peak trq max - Regen/1 -> Switch1/3
  Cont trq max - Regen/1 -> Switch/3
  Cont trq max - Motoring/1 -> Switch/1
  speed/1 -> rad/s  to RPM/1
  torque/1 -> Heat index/2(torque)
  Abs/1 -> Product5/2
  Sum/1 -> Abs/1, Sign/1
  Product5/1 -> max torque/1
  Sign/1 -> Product5/1
  Memory/1 -> Cont trq max - Motoring/1, Cont trq max - Regen/1, Peak trq max - Motoring1/1, Peak trq max - Regen/1
  rad/s  to RPM/1 -> Memory/1
  Constant/1 -> Divide/1
  RPM to rad/s/1 -> Divide by zero/1(In1)
  Abs2/1 -> 2-D Lookup Table/2
  Abs1/1 -> 2-D Lookup Table/1
  2-D Lookup Table/1 -> Gain2/1
  Gain2/1 -> Divide/2
  Req/1 -> Switch/2, Switch1/2
  Divide by zero/1(Out1) -> Divide/3
  Peak trq max - Motoring1/1 -> Switch1/1

== system P2_SIL_Model_Diag/Camaro Plant Model/On-Board Charger/Soft_OBC/NLG5_TEMP/NoiseAdd ==
  In : Inport
  Random Number : RandomNumber  Variance=variance  Seed=seed  SampleTime=tloop
  Rate Transition : RateTransition
  Sum : Sum  Inputs=|++
  Out : Outport
  wires:
  Sum/1 -> Out/1
  In/1 -> Sum/1
  Random Number/1 -> Rate Transition/1
  Rate Transition/1 -> Sum/2

== system P2_SIL_Model_Diag/Camaro Plant Model/On-Board Charger/Soft_OBC/NLG5_TEMP/NoiseAdd1 ==
  In : Inport
  Random Number : RandomNumber  Variance=variance  Seed=seed  SampleTime=tloop
  Rate Transition : RateTransition
  Sum : Sum  Inputs=|++
  Out : Outport
  wires:
  Rate Transition/1 -> Sum/2
  Random Number/1 -> Rate Transition/1
  In/1 -> Sum/1
  Sum/1 -> Out/1

== system P2_SIL_Model_Diag/Camaro Plant Model/On-Board Charger/Soft_OBC/NLG5_TEMP/NoiseAdd2 ==
  In : Inport
  Random Number : RandomNumber  Variance=variance  Seed=seed  SampleTime=tloop
  Rate Transition : RateTransition
  Sum : Sum  Inputs=|++
  Out : Outport
  wires:
  Sum/1 -> Out/1
  In/1 -> Sum/1
  Random Number/1 -> Rate Transition/1
  Rate Transition/1 -> Sum/2

== system P2_SIL_Model_Diag/Camaro Plant Model/Transmission1/Soft TCM/6L45 Logic/Gearbox_Control.Shift_Schedule.PlotShiftSchedule/Subsystem ==

== system P2_SIL_Model_Diag/Camaro Plant Model/Transmission1/Transmission Plant/Gearbox/Inertia Calculation ==
  Inertia_in : Inport
  gear number : Inport  Port=2
  Product2 : Product  Inputs=3  SaturateOnIntegerOverflow=on  InputSameDT=on  OutDataTypeStr=Inherit: Same as first input
  Sum : Sum  Inputs=|++  SaturateOnIntegerOverflow=on  InputSameDT=on  OutDataTypeStr=Inherit: Same as first input
  Sum2 : Sum  Inputs=|++  SaturateOnIntegerOverflow=on  InputSameDT=on  OutDataTypeStr=Inherit: Same as first input
  Switch : Switch  Criteria=u2 ~= 0  Threshold=0.5  SaturateOnIntegerOverflow=on  InputSameDT=on
  gb_inertia_in : Constant  Value=gb.plant.init.inertia_in
  gb_inertia_out : Constant  Value=gb.plant.init.inertia_out
  gear ratio table : Lookup  InputValues=gb.plant.init.ratio.idx1_gear  Table=gb.plant.init.ratio.map  OutDataTypeStr=double  SaturateOnIntegerOverflow=on
  Inertia : Outport
  wires:
  gear ratio table/1 -> Product2/1, Product2/2
  Sum2/1 -> Switch/1
  Inertia_in/1 -> Sum/1
  Product2/1 -> Sum2/1
  gb_inertia_in/1 -> Sum/2
  Sum/1 -> Product2/3
  gb_inertia_out/1 -> Sum2/2, Switch/3
  gear number/1 -> Switch/2, gear ratio table/1
  Switch/1 -> Inertia/1

== system P2_SIL_Model_Diag/Camaro Plant Model/Transmission1/Transmission Plant/Gearbox/Speed Calculation ==
  gear number : Inport
  spd out : Inport  Port=2
  torque input : Inport  Port=3
  Inertia Input : Inport  Port=4
  Fcn2 : Fcn  Expr=(u[1]==0)*u[4]+(u[1]==1)*u[2]+(u[1]>1)*u[3]
  Mux : Mux
  P/N : Subsystem
  Product : Product  SaturateOnIntegerOverflow=on  InputSameDT=on  OutDataTypeStr=Inherit: Same as first input
  R/D : Subsystem
  gear ratio table : Lookup  InputValues=gb.plant.init.ratio.idx1_gear  Table=gb.plant.init.ratio.map  SaturateOnIntegerOverflow=on
  Speed : Outport
  wires:
  Mux/1 -> Fcn2/1
  Fcn2/1 -> Speed/1
  P/N/1(speed) -> Mux/4
  R/D/1(spd in filtered) -> Mux/3
  gear number/1 -> Mux/1, P/N/3(gear), R/D/2(gear number), gear ratio table/1
  torque input/1 -> P/N/1(torque input)
  Inertia Input/1 -> P/N/2(Inertia Input)
  spd out/1 -> Product/1
  gear ratio table/1 -> Product/2
  Product/1 -> Mux/2, R/D/1(spd in), P/N/4(inital speed)

== system P2_SIL_Model_Diag/Camaro Plant Model/Transmission1/Transmission Plant/Gearbox/Torque calculation ==
  speed out : Inport
  gear number : Inport  Port=2
  " input torque" : Inport  Port=3
  Abs : Abs  SaturateOnIntegerOverflow=on
  Abs1 : Abs  SaturateOnIntegerOverflow=on
  Blending (state dependent) : Subsystem  mask(State dependent blending){xl=-gb.plant.init.spd_thr, yl=-1, xc=0, yc=0, xr=gb.plant.init.spd_thr, yr=1}
      mask prompts: xl "Left point (x):"; yl "Left point (y):"; xc "Center point (x):"; yc "Center point (y):"; xr "Right point (x):"; yr "Right point (y):"
      mask help: This block implements state dependent smoothing/blending. IMPORTANT: See help menu.
      mask Help: The output equals the product of the first input and a "hat" function defined by the three points specified in the dialog box.  The second input forms the argument to the hat function.\n\nIMPORTANT: A divide by zero error will result if first coordinates of the three points specified for the hat function are NOT distinct.
      mask Display: plot([-1 1 3 6 8], [1.5 1.5 0.5 4.0 4.0])
  Product5 : Product  SaturateOnIntegerOverflow=on  InputSameDT=on  OutDataTypeStr=Inherit: Same as first input
  Product6 : Product  SaturateOnIntegerOverflow=on  InputSameDT=on  OutDataTypeStr=Inherit: Same as first input
  Saturation1 : Saturate  UpperLimit=inf  LowerLimit=min( gb.plant.init.trq_loss.idx1_trq )
  Saturation2 : Saturate  UpperLimit=inf  LowerLimit=min( gb.plant.init.trq_loss.idx2_spd )
  Sum1 : Sum  Inputs=+-  SaturateOnIntegerOverflow=on  InputSameDT=on  OutDataTypeStr=Inherit: Same as first input
  Torque loss : Lookup_n-D  NumberOfTableDimensions=3  BreakpointsForDimension1=gb.plant.init.trq_loss.idx1_trq  BreakpointsForDimension2=gb.plant.init.trq_loss.idx2_spd  BreakpointsForDimension3=gb.plant.init.trq_loss.idx3_gear  Table=gb.plant.init.trq_loss.map
  gear ratio table : Lookup  InputValues=gb.plant.init.ratio.idx1_gear  Table=gb.plant.init.ratio.map  SaturateOnIntegerOverflow=on
  torque_out : Outport
  wires:
  Saturation2/1 -> Torque loss/2
  Saturation1/1 -> Torque loss/1
  Abs/1 -> Saturation1/1
  gear ratio table/1 -> Product5/2, Product6/1
  Product5/1 -> Abs1/1, Blending (state dependent)/2(Control (state))  "dtr_trans_speed"
  Abs1/1 -> Saturation2/1
  speed out/1 -> Product5/1
  Product6/1 -> torque_out/1
  Blending (state dependent)/1(Output) -> Sum1/2
  Sum1/1 -> Product6/2
  Torque loss/1 -> Blending (state dependent)/1(Input)
  " input torque"/1 -> Sum1/1, Abs/1
  gear number/1 -> Torque loss/3, gear ratio table/1

== system P2_SIL_Model_Diag/Camaro Plant Model/Transmission1/Transmission Plant/Torque Converter/Inertia Calculation ==
  inertia in : Inport
  lockup cmd : Inport  Port=2
  Pump Inertia : Constant  Value=tc.plant.init.inertia_in
  Sum2 : Sum  SaturateOnIntegerOverflow=on  InputSameDT=on  OutDataTypeStr=Inherit: Same as first input
  Sum5 : Sum  Inputs=|++  SaturateOnIntegerOverflow=on  InputSameDT=on  OutDataTypeStr=Inherit: Same as first input
  Switch2 : Switch  Threshold=eps  SaturateOnIntegerOverflow=on  InputSameDT=on
  Turbine Inertia : Constant  Value=tc.plant.init.inertia_out
  turbine inertia : Outport
  impeller inertia : Outport  Port=2
  wires:
  Sum5/1 -> Switch2/1
  lockup cmd/1 -> Switch2/2
  Switch2/1 -> turbine inertia/1
  Pump Inertia/1 -> Sum2/2
  Sum2/1 -> Sum5/1, impeller inertia/1
  Turbine Inertia/1 -> Switch2/3, Sum5/2
  inertia in/1 -> Sum2/1

== system P2_SIL_Model_Diag/Camaro Plant Model/Transmission1/Transmission Plant/Torque Converter/Speed Calculation ==
  turbine_spd : Inport
  impeller_inertia : Inport  Port=2
  lockup_cmd : Inport  Port=3
  impeller_trq : Inport  Port=4
  Memory : Memory
  Only Positive : Saturate  UpperLimit=inf  LowerLimit=0
  Pump Accel : Subsystem  mask(Division){}
      mask Display: disp('/')
  Slip speed integrator : Subsystem  mask(Resettable integrator){init=tc.plant.init.spd_idle}
      mask prompts: init "Initial value:"
      mask help: Integrates first input. If second input is not zero, integration stops and state is set to third input.
      mask Help: RESETTABLE INTEGRATOR  The resettable integrator is a masked function. This block has same functionality as the built-in RESET INTEGRATOR except that when input 2 is non-zero, the block stops integration.
  impeller spd : Outport
  wires:
  impeller_trq/1 -> Pump Accel/2(x)
  turbine_spd/1 -> Slip speed integrator/3(Reset value)
  lockup_cmd/1 -> Slip speed integrator/2(Control)
  Pump Accel/1(x\y) -> Slip speed integrator/1(Integral)  "alpha"
  impeller_inertia/1 -> Pump Accel/1(y)
  Slip speed integrator/1(Output) -> Only Positive/1
  Only Positive/1 -> Memory/1
  Memory/1 -> impeller spd/1

== system P2_SIL_Model_Diag/Camaro Plant Model/Transmission1/Transmission Plant/Torque Converter/Torque Calculation ==
  "impeller_spd " : Inport
  turbine_spd : Inport  Port=2
  lockup_cmd : Inport  Port=3
  input_trq : Inport  Port=4
  " Hydraulic Dynamic Torque" : Subsystem
  Switch : Switch  Threshold=1
  spd and trq ratio : Subsystem
  "impeller_trq " : Outport
  turbine_trq : Outport  Port=2
  wires:
  lockup_cmd/1 -> Switch/2
  Switch/1 -> turbine_trq/1
  input_trq/1 -> " Hydraulic Dynamic Torque"/1(input_trq), Switch/1
  " Hydraulic Dynamic Torque"/1(turbine_trq) -> Switch/3
  spd and trq ratio/1(Rt) -> " Hydraulic Dynamic Torque"/2(Rt)
  " Hydraulic Dynamic Torque"/2(impeller_trq) -> "impeller_trq "/1
  spd and trq ratio/2(Rw) -> " Hydraulic Dynamic Torque"/3(Rw)
  "impeller_spd "/1 -> " Hydraulic Dynamic Torque"/4(impeller_spd), spd and trq ratio/1(impeller spd)
  turbine_spd/1 -> spd and trq ratio/2(turbine spd)

== system P2_SIL_Model_Diag/Controller/HSC/Camaro Fault Detection/Component Diagnostic/Clutch Component Diagnostic ==
  In1 : Inport
  Bus Creator1 : BusCreator  Inputs=1
  Bus Selector : BusSelector  OutputSignals=Clutch_SigDiag.ClutchRollingAliveActive,Clutch_SigDiag.Engage_Clutch_SigValid,Clutch_SigDiag.clt_plant_spd_out_SigValid,Clutch_SigDiag.Engage_Failed
  Clutch_CompDia : Stateflow chart  TreatAsAtomicUnit=on
  Out1 : Outport
  wires:
  In1/1 -> Bus Selector/1
  Bus Creator1/1 -> Out1/1
  Bus Selector/1 -> Clutch_CompDia/1(ClutchRollingAliveActive_SigValid)  "<ClutchRollingAliveActive>"
  Bus Selector/2 -> Clutch_CompDia/2(Engage_Clutch_SigValid)  "<Engage_Clutch_SigValid>"
  Bus Selector/3 -> Clutch_CompDia/3(clt_plant_spd_out_SigValid)  "<clt_plant_spd_out_SigValid>"
  Clutch_CompDia/1(Clutch_Status) -> Bus Creator1/1  "Clutch_Status"
  Bus Selector/4 -> Clutch_CompDia/4(EngageFailed)  "<Engage_Failed>"
